simulink model "Model"  (Simulink 8.0)
settings: Solver=ode3  StartTime=0.0  StopTime=20  FixedStep=0.1  RelTol=1e-3
InitFcn:
  | a=APRBS(1000,0.5,1.5,1)
libraries: dspsrcs4 x1
settings Model: Creator=Saman  LastModifiedBy=Saman

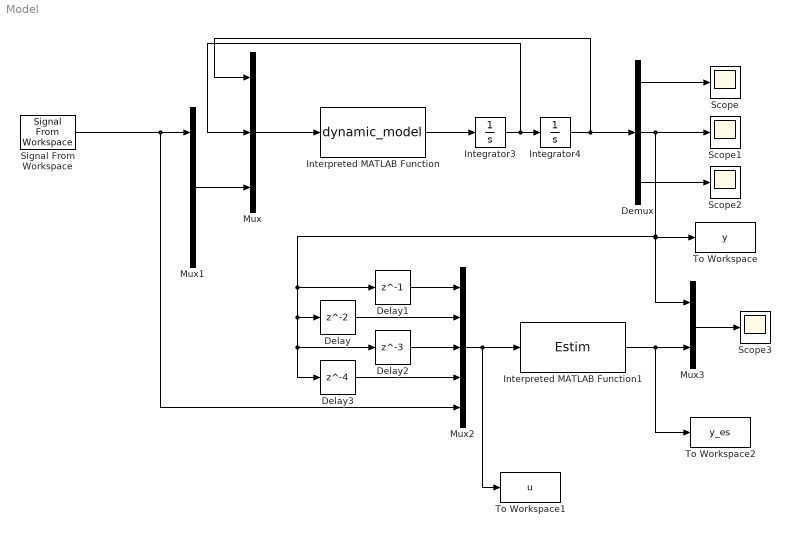
== system Model ==
  Delay : Delay  InitialCondition=0
  Delay1 : Delay  DelayLength=1  InitialCondition=0
  Delay2 : Delay  DelayLength=3  InitialCondition=0
  Delay3 : Delay  DelayLength=4  InitialCondition=0
  Demux : Demux  Outputs=3
  Integrator3 : Integrator  InitialCondition=[0;0;0]
  Integrator4 : Integrator  InitialCondition=[0;0;0]
  Interpreted MATLAB Function : MATLABFcn  MATLABFcn=dynamic_model  OutputDimensions=3
  Interpreted MATLAB Function1 : MATLABFcn  MATLABFcn=Estim  OutputDimensions=1  Output1D=off  SampleTime=0.1
  Mux : Mux  Inputs=3
  Mux1 : Mux  Inputs=3
  Mux2 : Mux  Inputs=5
  Mux3 : Mux  Inputs=2
  Scope{,1..3} (4 alike) : Scope
      Scope2 settings: SaveName=ScopeData2
      Scope3 settings: SaveName=ScopeData3
  Signal From Workspace : dspsrcs4/Signal From Workspace  X=a  Ts=0.1  nsamps=1  OutputAfterFinalValue=Setting to zero  ignoreOrWarnInputAndFrameLengths=off
  To Workspace : ToWorkspace  VariableName=y  SampleTime=0.1
  To Workspace1 : ToWorkspace  VariableName=u  SampleTime=0.1
  To Workspace2 : ToWorkspace  VariableName=y_es  SampleTime=0.1
  wires:
  Mux/1 -> Interpreted MATLAB Function/1
  Interpreted MATLAB Function/1 -> Integrator3/1
  Integrator3/1 -> Mux/2, Integrator4/1
  Mux1/1 -> Mux/3
  Signal From Workspace/1 -> Mux2/5, Mux1/1
  Integrator4/1 -> Demux/1, Mux/1
  Demux/1 -> Scope/1
  Demux/3 -> Scope2/1
  Delay/1 -> Mux2/2
  Delay1/1 -> Mux2/1
  Demux/2 -> Mux3/1, To Workspace/1, Delay1/1, Delay2/1, Delay3/1, Delay/1, Scope1/1
  Interpreted MATLAB Function1/1 -> To Workspace2/1, Mux3/2
  Mux3/1 -> Scope3/1
  Mux2/1 -> Interpreted MATLAB Function1/1, To Workspace1/1
  Delay2/1 -> Mux2/3
  Delay3/1 -> Mux2/4
